simulink model "Main_Sim"  (R2018b)
settings: Solver=FixedStepAuto  StartTime=0.0  StopTime=5600  FixedStep=simParams.sample_time_s  RelTol=1e-3  EnableMultiTasking=on
undefined symbols (not defined in the file): simParams
libraries: actuators_lib x1, CDH_command_lib x1, Environment_lib x1, FSW_Lib x1, Sensors_Lib x1, quat_degerr_lib x1, satelliteDynamics_lib x1
settings Model: Creator=devantormey  LastModifiedBy=Taylor
settings OptimizationCC: DefaultParameterBehavior=Inlined  UseDivisionForNetSlopeComputation=on  UseFloatMulNetSlope=on  InlineInvariantSignals=on  PassReuseOutputArgsAs=Individual arguments  ZeroExternalMemoryAtStartup=off  ZeroInternalMemoryAtStartup=off  NoFixptDivByZeroProtection=on  EfficientFloat2IntCast=on  LifeSpan=1  OptimizeBlockOrder=speed  DifferentSizesBufferReuse=on
settings DebuggingCC: ParameterTunabilityLossMsg=error  BusObjectLabelMismatch=error  SFUnexpectedBacktrackingDiag=warning  SFNoUnconditionalDefaultTransitionDiag=warning
settings HardwareCC: ProdBitPerPointer=32  ProdBitPerSizeT=32  ProdBitPerPtrDiffT=32  ProdLargestAtomicInteger=Long  ProdLargestAtomicFloat=Double  ProdWordSize=32  ProdLongLongMode=on  ProdHWDeviceType=NXP->Cortex-M4
settings SFSimCC: SimUseLocalCustomCode=off  MATLABDynamicMemAlloc=off
settings RTWCC: SystemTargetFile=ert.tlc  TemplateMakefile=ert_default_tmf  GenerateReport=on  RTWUseLocalCustomCode=off  IncludeHyperlinkInReport=on  LaunchReport=on  GenerateTraceInfo=on  GenerateTraceReport=on  GenerateTraceReportSl=on  GenerateTraceReportSf=on  GenerateTraceReportEml=on  GenerateCodeMetricsReport=on
settings CodeAppCC: ForceParamTrailComments=on  IgnoreCustomStorageClasses=off  OperatorAnnotations=on  SimulinkDataObjDesc=on  SFDataObjDesc=on  CustomSymbolStrGlobalVar=rt$N$M  CustomSymbolStrType=$N$M  CustomSymbolStrFcn=$N$M$F  CustomSymbolStrMacro=$N$M  InsertBlockDesc=on
settings ERTTargetCC: GenerateSampleERTMain=on  IncludeMdlTerminateFcn=off  CombineSignalStateStructs=on  SupportComplex=off  SupportContinuousTime=on  SupportNonInlinedSFcns=on  InlinedParameterPlacement=NonHierarchical  ERTCustomFileTemplate=example_file_process.tlc
settings ConfigComp: CovMetricSettings=dw  CovHtmlReporting=on  CovSaveCumulativeToWorkspaceVar=on  CovSaveSingleToWorkspaceVar=on  CovExternalEMLEnable=off

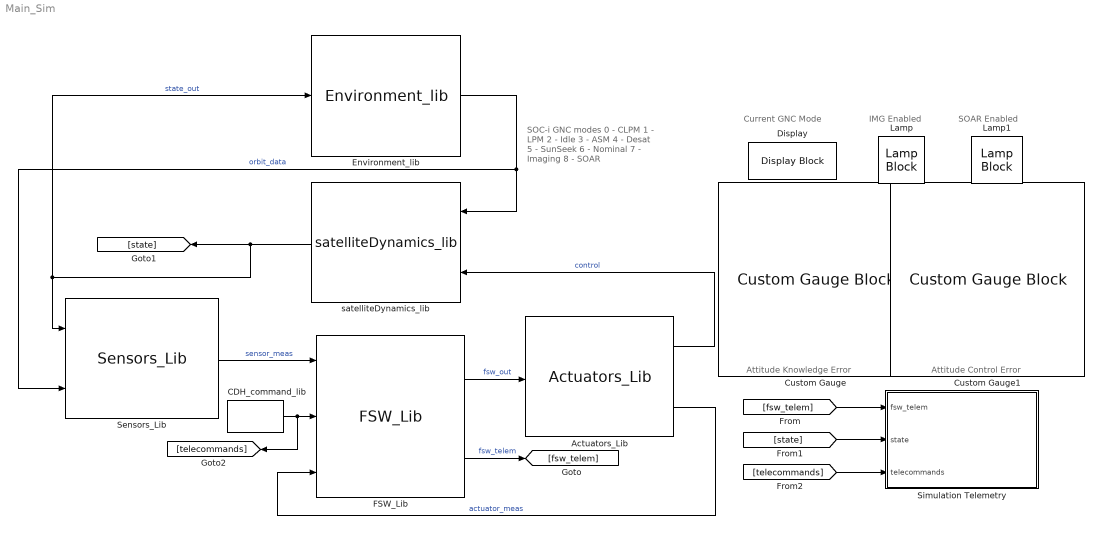
== system Main_Sim ==
  note: Attitude Knowledge Error
  note: SOC-i GNC modes
      | 0 - CLPM
      | 1 - LPM
      | 2 - Idle
      | 3 - ASM
      | 4 - Desat
      | 5 - SunSeek
      | 6 - Nominal
      | 7 - Imaging
      | 8 - SOAR
  note: Attitude Control Error
  note: Current GNC Mode
  note: IMG Enabled
  note: SOAR Enabled
  Actuators_Lib : actuators_lib/Actuators_Lib  SystemSampleTime=-1
  CDH_command_lib : CDH_command_lib/CDH_command_lib  target_lat_deg=target_lat_deg  target_lon_deg=target_lon_deg  target_alt_m=target_alt_m  override_autonomy=0  enable_pointing=on  force_clpm=off  force_lpm=off  enable_img=off  enable_soar=off  triad_override=off  MET_soar_utc_s=MET_soar_utc_s  quat_soar_cmd=quat_soar_cmd  mask{target_lat_deg=44.0, target_lon_deg=-76.5, target_alt_m=0.0, override_autonomy=0, enable_pointing=on, force_clpm=off, force_lpm=off, enable_img=off, enable_soar=off, triad_override=off, MET_soar_utc_s=simParams.time.epoch_utc_s+500, quat_soar_cmd=[0.200869388727445;-0.603600311719593;-0.740781711514794;-0.215779072779279]}
      mask prompts: target_lat_deg "Target Latitude [deg]"; target_lon_deg "Target Longitude [deg]"; target_alt_m "Target Alt [m]"; override_autonomy "Override Autonomous Mode Selection"; enable_pointing "Enable Autonomous Pointing"; force_clpm "CLPM Operating Mode"; force_lpm "LPM Operating Mode"; enable_img "Enable IMG"; enable_soar "Enable SOAR"; triad_override "TRIAD Override"; MET_soar_utc_s "SOARs MET Trigger"; quat_soar_cmd "SOARs Commanded Attitude"
      mask TypeOptions target_lat_deg: target_lat_deg
      mask TypeOptions target_lon_deg: target_lon_deg
      mask TypeOptions target_alt_m: target_alt_m
      mask TypeOptions override_autonomy: override_autonomy
      mask TypeOptions enable_pointing: enable_pointing
      mask TypeOptions force_clpm: force_clpm
      mask TypeOptions force_lpm: force_lpm
      mask TypeOptions enable_img: enable_img
      mask TypeOptions enable_soar: enable_soar
      mask TypeOptions triad_override: triad_override
      mask TypeOptions MET_soar_utc_s: MET_soar_utc_s
      mask TypeOptions quat_soar_cmd: quat_soar_cmd
      mask DialogControl DescGroupVar Prompt: SOC-i Telecommand Module
      mask DialogControl DescTextVar Prompt: Adjust the parameters that can enter the GNC flight software from the rest of the satellite, including the other subsystems onboard and those that come from the ground station.
  Custom Gauge : CustomGaugeBlock  WebBlockId=302  LabelPosition=Hide  NeedleImage=data:image/svg+xml;base64,PD94bWwgdmVyc2lvbj0iMS4wIiBlbmNvZGluZz0idXRmLTgiPz4KPCEtLSBHZW5lcmF0b3I6IEFkb2JlIElsbHVzdHJhdG9yIDE5LjIuMSwgU1ZHIEV4cG9ydCBQbHVnLUluIC4gU1ZHIFZlcnNpb246IDYuMDAgQnVpbGQgMCkgIC0tPgo8c3ZnIHZlcnNpb249IjEuMSIgeG1sbnM9Imh0dHA6Ly93d3cudzMub3JnLzIwMDAvc3ZnIiB4bWxuczp4bGluaz0iaHR0cDovL3d3dy53My5vcmcvMTk5OS94bGluayIgeD0iMHB4IiB5PSIwcHgiCgkgdmlld0JveD0iMCAwIDIwMCA1MCIgc3R5bGU9ImVuYWJsZS1iYWNrZ3JvdW5kOm5ldyAw ...(+9940 chars)  NeedleXPos=0.3802298124325669  NeedleYPos=0.48117305677424654  NeedleHeight=0.11602152693163792  NeedleWidth=0.1911368983686954  NeedleInitialRotation=-59.94322499147643  BackgroundImage=data:image/svg+xml;base64,PD94bWwgdmVyc2lvbj0iMS4wIiBlbmNvZGluZz0iVVRGLTgiIHN0YW5kYWxvbmU9Im5vIj8+CjwhLS0gR2VuZXJhdG9yOiBBZG9iZSBJbGx1c3RyYXRvciAxOS4yLjEsIFNWRyBFeHBvcnQgUGx1Zy1JbiAuIFNWRyBWZXJzaW9uOiA2LjAwIEJ1aWxkIDApICAtLT4KCjxzdmcKICAgeG1sbnM6ZGM9Imh0dHA6Ly9wdXJsLm9yZy9kYy9lbGVtZW50cy8xLjEvIgogICB4bWxuczpjYz0iaHR0cDovL2NyZWF0aXZlY29tbW9ucy5vcmcvbnMjIgogICB4bWxuczpyZGY9Imh0dHA6Ly93d3cudzMub3JnLzE5OTkvMDIvMjItcmRmLXN5bnRh ...(+9660 chars)  GaugeMax=10  GaugeArcDefined=true  GaugeArcRadius=0.1358563990074277  GaugeArcStrokeWidth=0.03972965542329953  GaugeArcRotation=240.5385250290321  GaugeArcRatio=0.8333333333333  GaugeArcTransparency=0  ValueArcColor=#1759b0  GaugeTickColor=#faf5c8  TickInterval=1  ScaleColorsJSON="[{\"Min\":0,\"Max\":1,\"Color\":[0.39215686274509803,0.83137254901960778,0.074509803921568626]},{\"Min\":1,\"Max\":3.5,\"Color\":[0.92941176470588238,0.69411764705882351,0.12549019607843137]},{\"Min\":3.5,\"Max\":10,\"Color\":[0.8901960784313725,0.090196078431372548,0.050980392156862744]}]"  fixedAspectRatio=on
  Custom Gauge1 : CustomGaugeBlock  WebBlockId=312  LabelPosition=Bottom  NeedleImage=data:image/svg+xml;base64,PD94bWwgdmVyc2lvbj0iMS4wIiBlbmNvZGluZz0idXRmLTgiPz4KPCEtLSBHZW5lcmF0b3I6IEFkb2JlIElsbHVzdHJhdG9yIDE5LjIuMSwgU1ZHIEV4cG9ydCBQbHVnLUluIC4gU1ZHIFZlcnNpb246IDYuMDAgQnVpbGQgMCkgIC0tPgo8c3ZnIHZlcnNpb249IjEuMSIgeG1sbnM9Imh0dHA6Ly93d3cudzMub3JnLzIwMDAvc3ZnIiB4bWxuczp4bGluaz0iaHR0cDovL3d3dy53My5vcmcvMTk5OS94bGluayIgeD0iMHB4IiB5PSIwcHgiCgkgdmlld0JveD0iMCAwIDIwMCA1MCIgc3R5bGU9ImVuYWJsZS1iYWNrZ3JvdW5kOm5ldyAw ...(+9940 chars)  NeedleXPos=0.3802298124325669  NeedleYPos=0.48117305677424654  NeedleHeight=0.11602152693163792  NeedleWidth=0.1911368983686954  NeedleInitialRotation=-59.94322499147643  BackgroundImage=data:image/svg+xml;base64,PD94bWwgdmVyc2lvbj0iMS4wIiBlbmNvZGluZz0iVVRGLTgiIHN0YW5kYWxvbmU9Im5vIj8+CjwhLS0gR2VuZXJhdG9yOiBBZG9iZSBJbGx1c3RyYXRvciAxOS4yLjEsIFNWRyBFeHBvcnQgUGx1Zy1JbiAuIFNWRyBWZXJzaW9uOiA2LjAwIEJ1aWxkIDApICAtLT4KCjxzdmcKICAgeG1sbnM6ZGM9Imh0dHA6Ly9wdXJsLm9yZy9kYy9lbGVtZW50cy8xLjEvIgogICB4bWxuczpjYz0iaHR0cDovL2NyZWF0aXZlY29tbW9ucy5vcmcvbnMjIgogICB4bWxuczpyZGY9Imh0dHA6Ly93d3cudzMub3JnLzE5OTkvMDIvMjItcmRmLXN5bnRh ...(+9660 chars)  GaugeMax=10  GaugeArcDefined=true  GaugeArcRadius=0.1358563990074277  GaugeArcStrokeWidth=0.03972965542329953  GaugeArcRotation=240.5385250290321  GaugeArcRatio=0.8333333333333  GaugeArcTransparency=0  ValueArcColor=#1759b0  GaugeTickColor=#faf5c8  TickInterval=1  ScaleColorsJSON="[{\"Min\":0,\"Max\":1,\"Color\":[0.39215686274509803,0.83137254901960778,0.074509803921568626]},{\"Min\":1,\"Max\":3.5,\"Color\":[0.92941176470588238,0.69411764705882351,0.12549019607843137]},{\"Min\":3.5,\"Max\":10,\"Color\":[0.8901960784313725,0.090196078431372548,0.050980392156862744]}]"  fixedAspectRatio=on
  Display : DisplayBlock  WebBlockId=320  LabelPosition=Hide
  Environment_lib : Environment_lib/Environment_lib  SystemSampleTime=-1
  FSW_Lib : FSW_Lib/FSW_Lib  SystemSampleTime=-1
  Lamp : LampBlock  WebBlockId=336  LabelPosition=Hide
  Lamp1 : LampBlock  WebBlockId=337  LabelPosition=Hide
  Sensors_Lib : Sensors_Lib/Sensors_Lib  SystemSampleTime=-1
  Simulation Telemetry : Subsystem
  satelliteDynamics_lib : satelliteDynamics_lib/satelliteDynamics_lib  SystemSampleTime=-1
  wires:
  FSW_Lib/1 -> Actuators_Lib/1  "fsw_out"
  Sensors_Lib/1 -> FSW_Lib/1  "sensor_meas"
  satelliteDynamics_lib/1 -> Environment_lib/1, Sensors_Lib/1, [state]  "state_out"
  Environment_lib/1 -> satelliteDynamics_lib/1, Sensors_Lib/2  "orbit_data"
  Actuators_Lib/1 -> satelliteDynamics_lib/2  "control"
  CDH_command_lib/1 -> [telecommands], FSW_Lib/2
  Actuators_Lib/2 -> FSW_Lib/3  "actuator_meas"
  FSW_Lib/2 -> [fsw_telem]  "fsw_telem"
  [fsw_telem] -> Simulation Telemetry/1(fsw_telem)
  [state] -> Simulation Telemetry/2(state)
  [telecommands] -> Simulation Telemetry/3(telecommands)

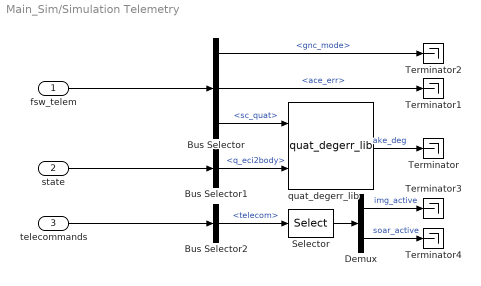
== system Main_Sim/Simulation Telemetry ==
  fsw_telem : Inport
  state : Inport  Port=2
  telecommands : Inport  Port=3
  Bus Selector : BusSelector  OutputSignals=gnc_mode,ace_err,sc_quat
  Bus Selector1 : BusSelector  OutputSignals=q_eci2body
  Bus Selector2 : BusSelector  OutputSignals=telecom
  Demux : Demux  Outputs=2
  Selector : Selector  InputPortWidth=6  IndexOptions=Index vector (dialog)  Indices=[5 6]  OutputSizes=1
  Terminator{,1..4} (5 alike) : Terminator
  quat_degerr_lib : quat_degerr_lib/quat_degerr_lib  SystemSampleTime=-1
  wires:
  telecommands/1 -> Bus Selector2/1
  quat_degerr_lib/1 -> Terminator/1  "ake_deg"
  Bus Selector1/1 -> quat_degerr_lib/2  "<q_eci2body>"
  fsw_telem/1 -> Bus Selector/1
  Selector/1 -> Demux/1
  Bus Selector2/1 -> Selector/1  "<telecom>"
  Bus Selector/1 -> Terminator2/1  "<gnc_mode>"
  Bus Selector/3 -> quat_degerr_lib/1  "<sc_quat>"
  Demux/2 -> Terminator4/1  "soar_active"
  Demux/1 -> Terminator3/1  "img_active"
  Bus Selector/2 -> Terminator1/1  "<ace_err>"
  state/1 -> Bus Selector1/1
